simulink model "Segvej_simulink"  (R2024a)
settings: Solver=VariableStepAuto  StartTime=0.0  StopTime=15  RelTol=1e-3
values from neighbouring files (symbols this model uses):
  A = [0        1                   0                  0 ... (first row only)    [segvej.m]
  a1 = a(1)    [segvej.m]
  a2 = a(2)    [segvej.m]
  a3 = a(3)    [segvej.m]
  a4 = a(4)    [segvej.m]
  B = [            0 ... (first row only)    [segvej.m]
  C = [1 0 0 0; 0 1 0 0; 0 0 1 0; 0 0 0 1]    [segvej.m]
  D = [0; 0; 0; 0]    [segvej.m]
  K = 1    [segvej.m]
  k1 = (M + m) * R + Iw / R    (= 773.25)    [segvej.m]
  k2 = m * l * R    (= 33.75)    [segvej.m]
  k3 = m * l    (= 225)    [segvej.m]
  k4 = Ir + m * l^2    (= 339.1875)    [segvej.m]
  k5 = m * l * g    (= 2207.25)    [segvej.m]
  k6 = M * l * R    (= 1.125)    [segvej.m]
settings Model: Creator=brati  LastModifiedBy=PC
settings RTWCC: GPUComputeCapability=3.5

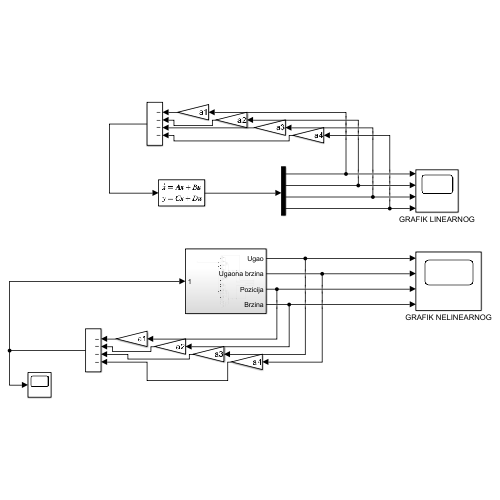
[thumbnail: Simulink's stored preview of the top-level diagram]
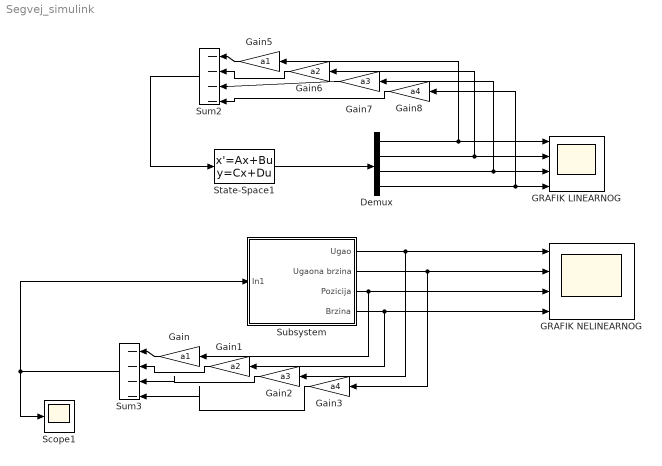
== system Segvej_simulink ==
  Demux : Demux
  GRAFIK LINEARNOG : Scope  NumInputPorts=4
  GRAFIK NELINEARNOG : Scope  NumInputPorts=4
  Gain : Gain  Gain=a1
  Gain1 : Gain  Gain=a2
  Gain2 : Gain  Gain=a3
  Gain3 : Gain  Gain=a4
  Gain5 : Gain  Gain=a1
  Gain6 : Gain  Gain=a2
  Gain7 : Gain  Gain=a3
  Gain8 : Gain  Gain=a4
  Scope1 : Scope
  State-Space1 : StateSpace  A=A  B=B  C=C  D=D  InitialCondition=[0 0 1 0]
  Subsystem : Subsystem
  Sum2 : Sum  Inputs=|-|-|-|-|
  Sum3 : Sum  Inputs=|-|-|-|-|
  wires:
  Subsystem/1(Ugao) -> Gain2/1, GRAFIK NELINEARNOG/1
  Subsystem/2(Ugaona brzina) -> Gain3/1, GRAFIK NELINEARNOG/2
  Subsystem/3(Pozicija) -> Gain/1, GRAFIK NELINEARNOG/3
  Subsystem/4(Brzina) -> Gain1/1, GRAFIK NELINEARNOG/4
  Gain/1 -> Sum3/1
  Gain1/1 -> Sum3/2
  Gain2/1 -> Sum3/3
  Gain3/1 -> Sum3/4
  State-Space1/1 -> Demux/1
  Demux/1 -> Gain5/1, GRAFIK LINEARNOG/1
  Demux/2 -> Gain6/1, GRAFIK LINEARNOG/2
  Demux/3 -> Gain7/1, GRAFIK LINEARNOG/3
  Demux/4 -> Gain8/1, GRAFIK LINEARNOG/4
  Gain5/1 -> Sum2/1
  Gain7/1 -> Sum2/3
  Gain8/1 -> Sum2/4
  Gain6/1 -> Sum2/2
  Sum3/1 -> Subsystem/1(In1), Scope1/1
  Sum2/1 -> State-Space1/1

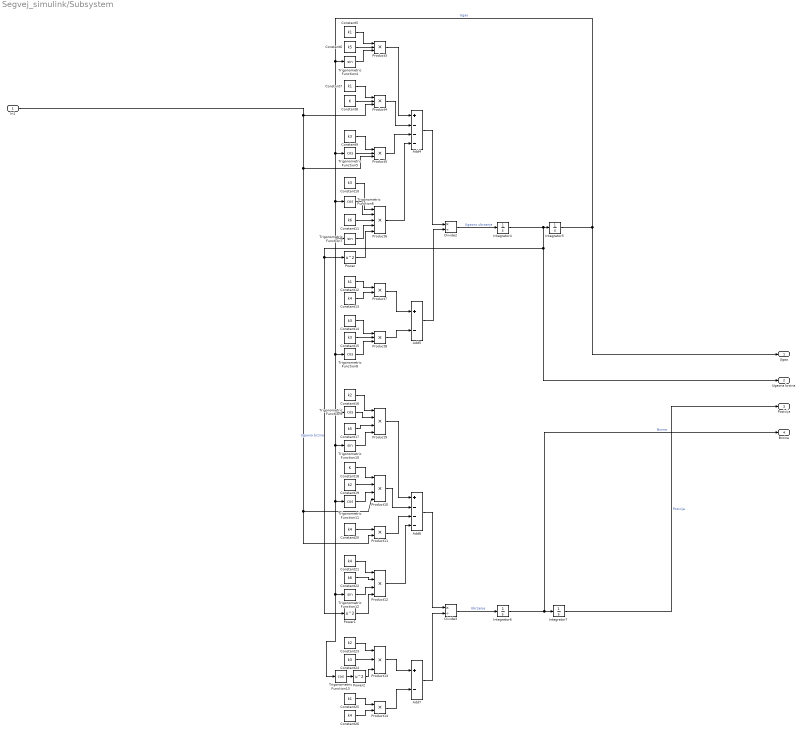
== system Segvej_simulink/Subsystem ==
  In1 : Inport
  Add4 : Sum  Inputs=+---
  Add5 : Sum  Inputs=+-
  Add6 : Sum  Inputs=+---
  Add7 : Sum  Inputs=+-
  Constant{9..10,14..15,24} (5 alike) : Constant  Value=k3
  Constant11 : Constant  Value=k6
  Constant{5,7,12,25} (4 alike) : Constant  Value=k1
  Constant{13,20..21,26} (4 alike) : Constant  Value=k4
  Constant16 : Constant  Value=k2
  Constant17 : Constant  Value=k5
  Constant18 : Constant  Value=K
  Constant19 : Constant  Value=k2
  Constant22 : Constant  Value=k6
  Constant23 : Constant  Value=k2
  Constant6 : Constant  Value=k5
  Constant8 : Constant  Value=K
  Divide2 : Product  Inputs=*/
  Divide3 : Product  Inputs=*/
  Integrator4 : Integrator
  Integrator5 : Integrator  InitialCondition=1
  Integrator6 : Integrator
  Integrator7 : Integrator
  Power : Math  Operator=square
  Power1 : Math  Operator=square
  Power2 : Math  Operator=square
  Product10 : Product  Inputs=4
  Product11 : Product
  Product12 : Product  Inputs=4
  Product{3..5,8,13} (5 alike) : Product  Inputs=3
  Product14 : Product
  Product6 : Product  Inputs=5
  Product7 : Product
  Product9 : Product  Inputs=4
  Trigonometric Function{4,7,10,12} (4 alike) : Trigonometry
  Trigonometric Function{5..6,8..9,11,13} (6 alike) : Trigonometry  Operator=cos
  Ugao : Outport
  Ugaona brzina : Outport  Port=2
  Pozicija : Outport  Port=3
  Brzina : Outport  Port=4
  wires:
  Constant15/1 -> Product8/2
  Integrator5/1 -> Ugao/1, Trigonometric Function4/1, Trigonometric Function9/1, Trigonometric Function13/1, Trigonometric Function12/1, Trigonometric Function11/1, Trigonometric Function10/1, Trigonometric Function8/1, Trigonometric Function7/1, Trigonometric Function6/1, Trigonometric Function5/1  "Ugao"
  In1/1 -> Product5/3, Product10/4, Product11/2, Product4/3
  Product3/1 -> Add4/1
  Constant20/1 -> Product11/1
  Constant19/1 -> Product10/2
  Integrator4/1 -> Ugaona brzina/1, Power/1, Power1/1, Integrator5/1  "Ugaona brzina"
  Trigonometric Function5/1 -> Product5/2
  Trigonometric Function10/1 -> Product9/4
  Trigonometric Function7/1 -> Product6/4
  Trigonometric Function8/1 -> Product8/3
  Product10/1 -> Add6/2
  Constant5/1 -> Product3/1
  Constant11/1 -> Product6/3
  Constant22/1 -> Product12/2
  Product4/1 -> Add4/2
  Constant26/1 -> Product14/2
  Constant25/1 -> Product14/1
  Constant10/1 -> Product6/1
  Product5/1 -> Add4/3
  Trigonometric Function13/1 -> Power2/1
  Product6/1 -> Add4/4
  Power2/1 -> Product13/3
  Add5/1 -> Divide2/2
  Constant18/1 -> Product10/1
  Trigonometric Function6/1 -> Product6/2
  Constant17/1 -> Product9/3
  Product8/1 -> Add5/2
  Constant24/1 -> Product13/2
  Constant6/1 -> Product3/2
  Trigonometric Function9/1 -> Product9/2
  Constant13/1 -> Product7/2
  Divide2/1 -> Integrator4/1  "Ugaono ubrzanje"
  Constant7/1 -> Product4/1
  Constant16/1 -> Product9/1
  Trigonometric Function4/1 -> Product3/3
  Product7/1 -> Add5/1
  Add4/1 -> Divide2/1
  Product9/1 -> Add6/1
  Power/1 -> Product6/5
  Constant8/1 -> Product4/2
  Constant23/1 -> Product13/1
  Trigonometric Function11/1 -> Product10/3
  Product12/1 -> Add6/4
  Product11/1 -> Add6/3
  Constant12/1 -> Product7/1
  Add6/1 -> Divide3/1
  Constant21/1 -> Product12/1
  Product14/1 -> Add7/2
  Power1/1 -> Product12/4
  Constant9/1 -> Product5/1
  Divide3/1 -> Integrator6/1  "Ubrzanje"
  Add7/1 -> Divide3/2
  Constant14/1 -> Product8/1
  Product13/1 -> Add7/1
  Integrator6/1 -> Brzina/1, Integrator7/1  "Brzina"
  Trigonometric Function12/1 -> Product12/3
  Integrator7/1 -> Pozicija/1  "Pozicija"
